simulink model "attempt_2_Full_Microthruster_Simulation"  (R2021b)
settings: Solver=ode45  StartTime=0.0  StopTime=simtime  RelTol=1e-16  AbsTol=1e-16
undefined symbols (not defined in the file): delta_t, dev_en, drag_unmodeled, dtype_g, euler_b_ECI0, euler_b_LVLH0, euler_LVLH_ECI0, g_bias, g_sath, g_satl, g_sen, g_sf_cc, geom, gr_eff_unmodeled, grav_grad_unmodeled, gyro_meas_frequ, J, JD_start, mag_field_unmodeled, mag_meas_frequ, mu, onboard_unmodeled, quat_b_ECI0, quat_b_LVLH0, quat_LVLH_ECI0, r, sigma_g, sigma_m, sigma_q, sigma_s, srp_unmodeled, sun_meas_frequ, theor_torque, ts, v, w_b_ECI0, wn, zn
libraries: aerolibnav x5, sharedTrackingLibrary x2
(part 2 of 2)

== matlab function attempt_2_Full_Microthruster_Simulation/Mag Sensor Measurement Function/MATLAB Function ==
  data: xk input; yy output; start_time input; sim_time input; sigma_m input; sigma_q input; posState input
function yy = h(xk,start_time,sim_time,sigma_m,sigma_q,posState)

yy = zeros([3 1]);
% Start time is initial juliandate
% Sim time is current sim time in seconds

JD_new = start_time + sim_time/3600/24; % add sim time in days to start time
t1 = datetime(JD_new,'ConvertFrom','juliandate');

q = xk(4:7);
eps = q(1:3);
eta = q(4);
r_ECI = posState(1:3);
[y, m, d] = ymd(t1);
[h, mm, s] = hms(t1);
utc_t1 = [y m d h mm s];
coder.extrinsic('eci2lla');
coder.extrinsic('igrfmagm');
coder.extrinsic('ned2ecefv');
coder.extrinsic('dcmeci2ecef');
coder.extrinsic('randn');
coder.extrinsic('decyear');

coder.extrinsic('Functions.Yb_func')
lla = eci2lla((r_ECI.*1e3)',utc_t1);
del = lla(1); % latitude
lambda = lla(2); % longitude
alt_g = lla(3);

% t = sim_time;
% % Set constants
% Re = 6378e3;                        % radius of the earth in m
% w_earth = 7.292e-5;                 % rad/s Earth rotation
% r_ECI_mag = norm(1e3.*r_ECI);       % magnitude of r ECI vector 
% m_b = [0;0;-0.5];                   % Residual magnetic dipole in body frame in A-m^2
% g1 = -29404.8*10^-9;                      % IGRF coeff constants
% g11 = -1450.9*10^-9;
% h11 = 4652.5*10^-9;

% Set intial conditions
% t0 = 0;                             % initial time

% Calculate B in BODY FRAME
% del = asin(r_ECI(3)/r_ECI_mag);     % geocentric latitude
% theta = pi/2 - del;                 % s/c geocentric co-latitude
% alpha = atan2((r_ECI(2)/sqrt(r_ECI(1)^2+r_ECI(2)^2)),... % s/c right ascension
%               (r_ECI(1)/sqrt(r_ECI(1)^2+r_ECI(2)^2))); 
% alpha_G = w_earth*(t-t0);           % right ascension of Greenwich meridian
% lambda = alpha - alpha_G;           % s/c geocentric longitude 
% C_ECI_s = Functions.Cz(-alpha)*Functions.Cy(del-pi/2);  % rotation matrix from spherical to ECI
% 
% mag_ECI = C_ECI_s*[2*(Re/r_ECI_mag)^3*(g1*cos(theta) + (g11*cos(lambda)+h11*sin(lambda))*sin(theta));
%          (Re/r_ECI_mag)^3*(g1*sin(theta) + (g11*cos(lambda)+h11*sin(lambda))*sin(theta));
%          (Re/r_ECI_mag)^3*(g11*sin(lambda) - h11*cos(lambda))]; % Earth magnetic field in spherical coordinates

igrf_m_NED = igrfmagm(alt_g,del,lambda,decyear(y,m,d))*1e-9;
igrf_m_ECEF = [0 0 0];
[igrf_m_ECEF(1),igrf_m_ECEF(2),igrf_m_ECEF(3)] = ned2ecefv(igrf_m_NED(1),igrf_m_NED(2),igrf_m_NED(3),del,lambda);

C_ECEF_ECI = dcmeci2ecef('IAU-2000/2006',utc_t1);
C_ECI_ECEF = C_ECEF_ECI';
mag_ECI = C_ECI_ECEF*igrf_m_ECEF';

% Calculate Y(a,q) for magnetometer and sun sensor


Y_b = Functions.Yb_func(q,mag_ECI);

v_k = zeros([3 1]); %#ok<*PREALL> simulink needs this to determine variable size
v_k = randn(3,1)*sigma_q;   
m_k = zeros([3 1]);
m_k = randn(3,1)*sigma_m;
% y = [zeros(3) Y_s]*xk + m_k + v_k; % measurement with measurement and process noise
% y = [zeros(3) Y_s]*xk + mk + v_k; % measurement with measurement and process noise
yy = [zeros(3) Y_b]*xk; % measurement with no noise

== matlab function attempt_2_Full_Microthruster_Simulation/Magnetometer ==
  data: xk input; JD_start input; yy output; sigma_m input; sigma_q input; sim_time input; posState input; yy_no_noise output
function [yy,yy_no_noise] = magVec(xk,JD_start,sigma_m,sigma_q,sim_time,posState)

yy = zeros([3 1]);
JD_new = JD_start + sim_time/3600/24; % add sim time in days to start time
t1 = datetime(JD_new,'ConvertFrom','juliandate');

q = xk(4:7);

r_ECI = posState(1:3);

[y, m, d] = ymd(t1);
[h, mm, s] = hms(t1);
utc_t1 = [y m d h mm s];

coder.extrinsic('eci2lla');
coder.extrinsic('igrfmagm');
coder.extrinsic('ned2ecefv');
coder.extrinsic('dcmeci2ecef');
coder.extrinsic('randn');
coder.extrinsic('decyear');
coder.extrinsic('Functions.Yb_func')
lla = eci2lla((r_ECI.*1e3)',utc_t1);
del = lla(1); % latitude
lambda = lla(2); % longitude
alt_g = lla(3);

% Set constants
% Re = 6378e3;                        % radius of the earth in m
% w_earth = 7.292e-5;                 % rad/s Earth rotation
% r_ECI_mag = norm(1e3.*r_ECI);       % magnitude of r ECI vector 
% m_b = [0;0;-0.5];                   % Residual magnetic dipole in body frame in A-m^2
% g1 = -29404.8*10^-9;                      % IGRF coeff constants
% g11 = -1450.9*10^-9;
% h11 = 4652.5*10^-9;

% Set intial conditions
% t0 = 0;                             % initial time

% Calculate B in BODY FRAME
% del = asin(r_ECI(3)/r_ECI_mag);     % geocentric latitude
% theta = pi/2 - del;                 % s/c geocentric co-latitude
% alpha = atan2((r_ECI(2)/sqrt(r_ECI(1)^2+r_ECI(2)^2)),... % s/c right ascension
%               (r_ECI(1)/sqrt(r_ECI(1)^2+r_ECI(2)^2))); 
% alpha_G = w_earth*(t-t0);           % right ascension of Greenwich meridian
% lambda = alpha - alpha_G;           % s/c geocentric longitude 
% C_ECI_s = Functions.Cz(-alpha)*Functions.Cy(del-pi/2);  % rotation matrix from spherical to ECI
% 
% mag_ECI = C_ECI_s*[2*(Re/r_ECI_mag)^3*(g1*cos(theta) + (g11*cos(lambda)+h11*sin(lambda))*sin(theta));
%          (Re/r_ECI_mag)^3*(g1*sin(theta) + (g11*cos(lambda)+h11*sin(lambda))*sin(theta));
%          (Re/r_ECI_mag)^3*(g11*sin(lambda) - h11*cos(lambda))]; % Earth magnetic field in spherical coordinates

igrf_m_NED = igrfmagm(alt_g,del,lambda,decyear(y,m,d))*1e-9;
igrf_m_ECEF = [0 0 0];
[igrf_m_ECEF(1),igrf_m_ECEF(2),igrf_m_ECEF(3)] = ned2ecefv(igrf_m_NED(1),igrf_m_NED(2),igrf_m_NED(3),del,lambda);

C_ECEF_ECI = dcmeci2ecef('IAU-2000/2006',utc_t1);
C_ECI_ECEF = C_ECEF_ECI';
mag_ECI = [0;0;0];
mag_ECI = C_ECI_ECEF*igrf_m_ECEF';

% Calculate Y(a,q) for magnetometer and sun sensor
Y_b = zeros([3 4]);
Y_b = Functions.Yb_func(q,mag_ECI);
% Y_b = [eta*eye(3)-vec2cross(eps) -eps]*[Functions.vec2cross(mag_ECI) mag_ECI;
%                                                       -mag_ECI'                    0];
% Y_s = [eta*eye(3)-Functions.vec2cross(eps) -eps]*[Functions.vec2cross(sun_ECI) sun_ECI;
%                                                       -sun_ECI'                    0];

v_k = zeros([3 1]); %#ok<*PREALL> simulink needs this to determine variable size
v_k = randn(3,1)*sigma_q;   
m_k = zeros([3 1]);
m_k = [randn(3,1)*sigma_m];
yy_no_noise = [zeros(3) Y_b]*xk;
yy = yy_no_noise + m_k; % measurement with measurement and process noise
% y = [zeros(3) Y_s]*xk; % measurement with no noise

== matlab function attempt_2_Full_Microthruster_Simulation/State Transition Function/Perturbation Model 2/B Field/MATLAB Function ==
  data: state_rb input; Tmb output; attState input; t input
function Tmb = fcn(state_rb,attState,t)

%%% MAGNETIC FIELD %%%%%
r_ECI = state_rb(1:3)';
      
q = attState(4:end); % extract quaternion from attitude state
C_b_ECI = Functions.quat2rot(q); % get ECI to BODY rotation matrix % turn r_ECI into a column vector

% Set constants
Re = 6378e3;                        % radius of the earth in m
w_earth = 7.292e-5;                 % rad/s Earth rotation
r_ECI_mag = norm(1e3.*r_ECI);       % magnitude of r ECI vector 
m_b = [0;0;-0.5];                   % Residual magnetic dipole in body frame in A-m^2
g1 = -29404.8*10^-9;                      % IGRF coeff constants
g11 = -1450.9*10^-9;
h11 = 4652.5*10^-9;

% Set intial conditions
t0 = 0;                             % initial time

% Calculate B in BODY FRAME
del = asin(r_ECI(3)/r_ECI_mag);     % geocentric latitude
theta = pi/2 - del;                 % s/c geocentric co-latitude
alpha = atan2((r_ECI(2)/sqrt(r_ECI(1)^2+r_ECI(2)^2)),... % s/c right ascension
              (r_ECI(1)/sqrt(r_ECI(1)^2+r_ECI(2)^2))); 
alpha_G = w_earth*(t-t0);           % right ascension of Greenwich meridian
lambda = alpha - alpha_G;           % s/c geocentric longitude 
C_ECI_s = Functions.Cz(-alpha)*Functions.Cy(del-pi/2);  % rotation matrix from spherical to ECI

B_s = [2*(Re/r_ECI_mag)^3*(g1*cos(theta) + (g11*cos(lambda)+h11*sin(lambda))*sin(theta));
         (Re/r_ECI_mag)^3*(g1*sin(theta) + (g11*cos(lambda)+h11*sin(lambda))*sin(theta));
         (Re/r_ECI_mag)^3*(g11*sin(lambda) - h11*cos(lambda))]; % Earth magnetic field in spherical coordinates

B_b = C_b_ECI*C_ECI_s*B_s;          % Earth magnetic field in BODY frame
Tmb = [0;0;0];
Tmb = cross(m_b,B_b);               % magnetic field torque

== matlab function attempt_2_Full_Microthruster_Simulation/State Transition Function/Perturbation Model 2/Drag/MATLAB Function ==
  data: state input; Td output; attState input; geom input
function Td = fcn(state,attState,geom)

% Extract s/c geometry parameters
x = geom(1); % x-axis
y = geom(3); % y-axis
z = geom(2); % z-axis

v_ECI = state(4:6);
   
q = attState(4:end); % extract quaternion from attitude state
C_b_ECI = Functions.quat2rot(q);                 % get ECI to BODY rotation matrix 

%%%%%% ATMO DRAG %%%%%%%
v_b = 1000.*(C_b_ECI*v_ECI);    % velocity vector in BODY frame
v_mag = norm(v_b);      % velocity vector magnitude BODY frame
v_dir = v_b./v_mag;     % velocity unit vector BODY frame
Cd = 2.2;               % approximate coefficent of drag
rho = 1.49e-15;        % km/m^3 US std atmosphere


Ta = [0;0;0];                    % Initialzie atmo torque vector
Fd_coeff = -1/2*rho*v_mag^2*Cd;  % Calculate constant coeff for speed

% Instantiate CoP vectors
CoM_vec = [0;0;0]; % From mass_props inertia calculations; assume CoM is at center of body frame

%%%%%%%%%BUS COP VECTORS%%%%%%%%%%%%%%%%
BUS_neg_z = [0;0;-z/2];
CP_BUS_neg_z = CoM_vec - BUS_neg_z;

BUS_pos_z = -BUS_neg_z;
CP_BUS_pos_z = CoM_vec - BUS_pos_z;

BUS_neg_y = [0;-y/2;0];
CP_BUS_neg_y = CoM_vec - BUS_neg_y;

BUS_pos_y = -BUS_neg_y;
CP_BUS_pos_y = CoM_vec - BUS_pos_y;

BUS_neg_x = [-x/2;0;0];
CP_BUS_neg_x = CoM_vec - BUS_neg_x;

BUS_pos_x = -BUS_neg_x;
CP_BUS_pos_x = CoM_vec - BUS_pos_x;

% Find area of each exposed surface
A_SP_y_side = x*z;
A_SP_x_side = y*z;
A_SP_z_side = x*y;

% Create normal directional vectors
x_dir = [1;0;0];
y_dir = [0;1;0];
z_dir = [0;0;1];
dir_vector = {x_dir,-x_dir,y_dir,-y_dir,z_dir,-z_dir};

% Create arrays of areas and CoM-->CoP vectors for each surface for each
% normal direction (x, -x, y, -y, z, -z)
pos_x_COP_vectors = [CP_BUS_pos_x];
pos_x_areas       = [A_SP_x_side];

neg_x_areas        = pos_x_areas;
neg_x_COP_vectors = [CP_BUS_neg_x];

pos_y_COP_vectors = [CP_BUS_pos_y];
pos_y_areas        = [A_SP_y_side];

neg_y_areas        = pos_y_areas;
neg_y_COP_vectors = [CP_BUS_neg_y];

neg_z_areas        = [A_SP_z_side];
neg_z_COP_vectors = [CP_BUS_neg_z];

pos_z_areas        = [A_SP_z_side];
pos_z_COP_vectors = [CP_BUS_pos_z];

% Combine cell arrays of area and their corresponding vectors into parent
% cell arrays
CoP_vectors = {pos_x_COP_vectors,neg_x_COP_vectors,...
               pos_y_COP_vectors,neg_y_COP_vectors,...
               pos_z_COP_vectors,neg_z_COP_vectors};
areas = {pos_x_areas,neg_x_areas,pos_y_areas,neg_y_areas,pos_z_areas,neg_z_areas};

for i = 1:length(dir_vector)
    dire = dir_vector{i};
    if dot(dire,v_dir) >= 0
        curr_area = areas{i};
        curr_CoP_vec = CoP_vectors{i};
        for ii = 1:length(curr_area)
            Fd = dot(dire,v_dir)*Fd_coeff*curr_area(ii).*v_dir;
            Ta = Ta + cross(curr_CoP_vec(:,ii),Fd);
        end
    end
end

Td= Ta;

== matlab function attempt_2_Full_Microthruster_Simulation/State Transition Function/Perturbation Model 2/Gravity Gradient/MATLAB Function ==
  data: J input; Tgg output; state_rb input; attState input
function Tgg = fcn(J,state_rb,attState)

q = attState(4:end); % extract quaternion from attitude state

r_ECI = state_rb(1:3)*1000;
mu = 398600*1000^3;
   
C_b_ECI = Functions.quat2rot(q); % get ECI to BODY rotation matrix % turn r_ECI into a column vector
r_b = C_b_ECI*r_ECI;                        % Get r in terms of BODY frame
r_mag = norm(r_b);                          % Get magnitude of r in BODY frame
Tgg = (3*mu/r_mag^5)*Functions.vec2cross(r_b)*J*r_b; % Gravity gradient calculation

== matlab function attempt_2_Full_Microthruster_Simulation/State Transition Function/Perturbation Model 2/SRP/MATLAB Function ==
  data: attState input; Tsrp output; geom input
function Tsrp = fcn(attState,geom)


% Extract s/c geometry parameters
x = geom(1); % x-axis
y = geom(3); % y-axis
z = geom(2); % z-axis


q = attState(4:end); % extract quaternion from attitude state
C_b_ECI = Functions.quat2rot(q);                 % get ECI to BODY rotation matrix 
s_dir = C_b_ECI*[-1;0;0];     % solar radiation pressure unit vector BODY frame

%%%%%% ATMO DRAG %%%%%%%

% Instantiate CoP vectors
CoM_vec = [0;0;0]; % From mass_props inertia calculations; assume CoM is at center of body frame

%%%%%%%%%BUS COP VECTORS%%%%%%%%%%%%%%%%
BUS_neg_z = [0;0;-z/2];
CP_BUS_neg_z = CoM_vec - BUS_neg_z;

BUS_pos_z = -BUS_neg_z;
CP_BUS_pos_z = CoM_vec - BUS_pos_z;

BUS_neg_y = [0;-y/2;0];
CP_BUS_neg_y = CoM_vec - BUS_neg_y;

BUS_pos_y = -BUS_neg_y;
CP_BUS_pos_y = CoM_vec - BUS_pos_y;

BUS_neg_x = [-x/2;0;0];
CP_BUS_neg_x = CoM_vec - BUS_neg_x;

BUS_pos_x = -BUS_neg_x;
CP_BUS_pos_x = CoM_vec - BUS_pos_x;

% Find area of each exposed surface
A_SP_y_side = x*z;
A_SP_x_side = y*z;
A_SP_z_side = x*y;

% Create normal directional vectors
x_dir = [1;0;0];
y_dir = [0;1;0];
z_dir = [0;0;1];
dir_vector = {x_dir,-x_dir,y_dir,-y_dir,z_dir,-z_dir};

% Create arrays of areas and CoM-->CoP vectors for each surface for each
% normal direction (x, -x, y, -y, z, -z)
pos_x_COP_vectors = [CP_BUS_pos_x];
pos_x_areas       = [A_SP_x_side];

neg_x_areas        = pos_x_areas;
neg_x_COP_vectors = [CP_BUS_neg_x];

pos_y_COP_vectors = [CP_BUS_pos_y];
pos_y_areas        = [A_SP_y_side];

neg_y_areas        = pos_y_areas;
neg_y_COP_vectors = [CP_BUS_neg_y];

neg_z_areas        = [A_SP_z_side];
neg_z_COP_vectors = [CP_BUS_neg_z];

pos_z_areas        = [A_SP_z_side];
pos_z_COP_vectors = [CP_BUS_pos_z];

% Combine cell arrays of area and their corresponding vectors into parent
% cell arrays
CoP_vectors = {pos_x_COP_vectors,neg_x_COP_vectors,...
               pos_y_COP_vectors,neg_y_COP_vectors,...
               pos_z_COP_vectors,neg_z_COP_vectors};
areas = {pos_x_areas,neg_x_areas,pos_y_areas,neg_y_areas,pos_z_areas,neg_z_areas};

p_s = 4.5e-06; % solar const N/m^2
Tsrp = [0;0;0];                    % Initialzie atmo torque vector
for i = 1:length(dir_vector)
    dire = dir_vector{i};
    if dot(dire,s_dir) > 0
        curr_area = areas{i};
        curr_CoP_vec = CoP_vectors{i};
        for ii = 1:length(curr_area)
            Fs = -dot(dire,s_dir)*p_s*curr_area(ii).*s_dir;
            Tsrp = Tsrp + cross(curr_CoP_vec(:,ii),Fs);
        end
    end
end

== matlab function attempt_2_Full_Microthruster_Simulation/State Transition Function/MATLAB Function ==
  data: x_k_1 input; x_k output; u_k_1 input; T_thrust input; T_other input; J input; Ts input
function x_k = f(x_k_1,u_k_1,T_thrust,T_other,J,Ts)
% State transition function; propogating state (angular velocity and
% quaternion column vector) to new state via regular dynamic equations
% u_k_1 is some "control" value; set to 0 here
omega_k_1 = x_k_1(1:3);
quat_k_1 = x_k_1(4:7);

% Get last step b_ECI rotation matrix
C_b_ECI = Functions.quat2rot(quat_k_1);

% Turn given thrust vector from body to ECI
T_thrust = C_b_ECI'*T_thrust; % transpose b_ECI to get body->ECI rot matrix

T = T_thrust + T_other; % sum considered control/perturbation torques with applied thrust

eps = quat_k_1(1:3);
eta = quat_k_1(4);

x_k = x_k_1 + Ts*[J\(T-Functions.vec2cross(omega_k_1)*J*omega_k_1 + u_k_1);
                 0.5*(eta*eye(3)+Functions.vec2cross(eps))*omega_k_1;
                -0.5*eps'*omega_k_1];

== matlab function attempt_2_Full_Microthruster_Simulation/Mag Sensor Measurement Function1/MATLAB Function ==
  data: xk input; JD_start input; yy output; sim_time input; sigma_m input; sigma_q input; posState input
function yy = h(xk,JD_start,sim_time,sigma_m,sigma_q,posState)

% Start time is initial juliandate
% Sim time is current sim time in seconds

yy = zeros([3 1]);
JD_new = JD_start + sim_time/3600/24; % add sim time in days to start time
t1 = datetime(JD_new,'ConvertFrom','juliandate');

q = xk(4:7);
eps = q(1:3);
eta = q(4);
r_ECI = posState(1:3);
[y, m, d] = ymd(t1);
[h, mm, s] = hms(t1);
utc_t1 = [y m d h mm s];
coder.extrinsic('eci2lla');
coder.extrinsic('igrfmagm');
coder.extrinsic('ned2ecefv');
coder.extrinsic('dcmeci2ecef');
coder.extrinsic('randn');
coder.extrinsic('decyear');

coder.extrinsic('Functions.Yb_func')
lla = eci2lla((r_ECI.*1e3)',utc_t1);
del = lla(1); % latitude
lambda = lla(2); % longitude
alt_g = lla(3);

% t = sim_time;
% % Set constants
% Re = 6378e3;                        % radius of the earth in m
% w_earth = 7.292e-5;                 % rad/s Earth rotation
% r_ECI_mag = norm(1e3.*r_ECI);       % magnitude of r ECI vector 
% m_b = [0;0;-0.5];                   % Residual magnetic dipole in body frame in A-m^2
% g1 = -29404.8*10^-9;                      % IGRF coeff constants
% g11 = -1450.9*10^-9;
% h11 = 4652.5*10^-9;

% Set intial conditions
% t0 = 0;                             % initial time

% Calculate B in BODY FRAME
% del = asin(r_ECI(3)/r_ECI_mag);     % geocentric latitude
% theta = pi/2 - del;                 % s/c geocentric co-latitude
% alpha = atan2((r_ECI(2)/sqrt(r_ECI(1)^2+r_ECI(2)^2)),... % s/c right ascension
%               (r_ECI(1)/sqrt(r_ECI(1)^2+r_ECI(2)^2))); 
% alpha_G = w_earth*(t-t0);           % right ascension of Greenwich meridian
% lambda = alpha - alpha_G;           % s/c geocentric longitude 
% C_ECI_s = Functions.Cz(-alpha)*Functions.Cy(del-pi/2);  % rotation matrix from spherical to ECI
% 
% mag_ECI = C_ECI_s*[2*(Re/r_ECI_mag)^3*(g1*cos(theta) + (g11*cos(lambda)+h11*sin(lambda))*sin(theta));
%          (Re/r_ECI_mag)^3*(g1*sin(theta) + (g11*cos(lambda)+h11*sin(lambda))*sin(theta));
%          (Re/r_ECI_mag)^3*(g11*sin(lambda) - h11*cos(lambda))]; % Earth magnetic field in spherical coordinates

igrf_m_NED = igrfmagm(alt_g,del,lambda,decyear(y,m,d))*1e-9;
igrf_m_ECEF = [0 0 0];
[igrf_m_ECEF(1),igrf_m_ECEF(2),igrf_m_ECEF(3)] = ned2ecefv(igrf_m_NED(1),igrf_m_NED(2),igrf_m_NED(3),del,lambda);

C_ECEF_ECI = dcmeci2ecef('IAU-2000/2006',utc_t1);
C_ECI_ECEF = C_ECEF_ECI';
mag_ECI = C_ECI_ECEF*igrf_m_ECEF';

% Calculate Y(a,q) for magnetometer and sun sensor

Y_b = Functions.Yb_func(q,mag_ECI);

v_k = zeros([3 1]); %#ok<*PREALL> simulink needs this to determine variable size
v_k = randn(3,1)*sigma_q;   
m_k = zeros([3 1]);
m_k = randn(3,1)*sigma_m;
% y = [zeros(3) Y_s]*xk + m_k + v_k; % measurement with measurement and process noise
% y = [zeros(3) Y_s]*xk + mk + v_k; % measurement with measurement and process noise
yy = [zeros(3) Y_b]*xk; % measurement with no noise

== matlab function attempt_2_Full_Microthruster_Simulation/State Transition Function1/MATLAB Function ==
  data: x_k_1 input; x_k output; u_k_1 input; T_thrust input; T_other input; J input; Ts input
function x_k = f(x_k_1,u_k_1,T_thrust,T_other,J,Ts)
% State transition function; propogating state (angular velocity and
% quaternion column vector) to new state via regular dynamic equations
% u_k_1 is some "control" value; set to 0 here
omega_k_1 = x_k_1(1:3);
quat_k_1 = x_k_1(4:7);

% Get last step b_ECI rotation matrix
C_b_ECI = Functions.quat2rot(quat_k_1);

% Turn given thrust vector from body to ECI
T_thrust = C_b_ECI'*T_thrust; % transpose b_ECI to get body->ECI rot matrix

T = T_thrust + T_other; % sum considered control/perturbation torques with applied thrust

eps = quat_k_1(1:3);
eta = quat_k_1(4);

x_k = x_k_1 + Ts*[J\(T-Functions.vec2cross(omega_k_1)*J*omega_k_1 + u_k_1);
                 0.5*(eta*eye(3)+Functions.vec2cross(eps))*omega_k_1;
                -0.5*eps'*omega_k_1];

== matlab function attempt_2_Full_Microthruster_Simulation/State Transition Function1/Perturbation Model 2/B Field/MATLAB Function ==
  data: state_rb input; Tmb output; attState input; t input
function Tmb = fcn(state_rb,attState,t)

%%% MAGNETIC FIELD %%%%%
r_ECI = state_rb(1:3)';
      
q = attState(4:end); % extract quaternion from attitude state
C_b_ECI = Functions.quat2rot(q); % get ECI to BODY rotation matrix % turn r_ECI into a column vector

% Set constants
Re = 6378e3;                        % radius of the earth in m
w_earth = 7.292e-5;                 % rad/s Earth rotation
r_ECI_mag = norm(1e3.*r_ECI);       % magnitude of r ECI vector 
m_b = [0;0;-0.5];                   % Residual magnetic dipole in body frame in A-m^2
g1 = -29404.8*10^-9;                      % IGRF coeff constants
g11 = -1450.9*10^-9;
h11 = 4652.5*10^-9;

% Set intial conditions
t0 = 0;                             % initial time

% Calculate B in BODY FRAME
del = asin(r_ECI(3)/r_ECI_mag);     % geocentric latitude
theta = pi/2 - del;                 % s/c geocentric co-latitude
alpha = atan2((r_ECI(2)/sqrt(r_ECI(1)^2+r_ECI(2)^2)),... % s/c right ascension
              (r_ECI(1)/sqrt(r_ECI(1)^2+r_ECI(2)^2))); 
alpha_G = w_earth*(t-t0);           % right ascension of Greenwich meridian
lambda = alpha - alpha_G;           % s/c geocentric longitude 
C_ECI_s = Functions.Cz(-alpha)*Functions.Cy(del-pi/2);  % rotation matrix from spherical to ECI

B_s = [2*(Re/r_ECI_mag)^3*(g1*cos(theta) + (g11*cos(lambda)+h11*sin(lambda))*sin(theta));
         (Re/r_ECI_mag)^3*(g1*sin(theta) + (g11*cos(lambda)+h11*sin(lambda))*sin(theta));
         (Re/r_ECI_mag)^3*(g11*sin(lambda) - h11*cos(lambda))]; % Earth magnetic field in spherical coordinates

B_b = C_b_ECI*C_ECI_s*B_s;          % Earth magnetic field in BODY frame
Tmb = [0;0;0];
Tmb = cross(m_b,B_b);               % magnetic field torque

== matlab function attempt_2_Full_Microthruster_Simulation/State Transition Function1/Perturbation Model 2/Drag/MATLAB Function ==
  data: state input; Td output; attState input; geom input
function Td = fcn(state,attState,geom)

% Extract s/c geometry parameters
x = geom(1); % x-axis
y = geom(3); % y-axis
z = geom(2); % z-axis

v_ECI = state(4:6);
   
q = attState(4:end); % extract quaternion from attitude state
C_b_ECI = Functions.quat2rot(q);                 % get ECI to BODY rotation matrix 

%%%%%% ATMO DRAG %%%%%%%
v_b = 1000.*(C_b_ECI*v_ECI);    % velocity vector in BODY frame
v_mag = norm(v_b);      % velocity vector magnitude BODY frame
v_dir = v_b./v_mag;     % velocity unit vector BODY frame
Cd = 2.2;               % approximate coefficent of drag
rho = 1.49e-15;        % km/m^3 US std atmosphere


Ta = [0;0;0];                    % Initialzie atmo torque vector
Fd_coeff = -1/2*rho*v_mag^2*Cd;  % Calculate constant coeff for speed

% Instantiate CoP vectors
CoM_vec = [0;0;0]; % From mass_props inertia calculations; assume CoM is at center of body frame

%%%%%%%%%BUS COP VECTORS%%%%%%%%%%%%%%%%
BUS_neg_z = [0;0;-z/2];
CP_BUS_neg_z = CoM_vec - BUS_neg_z;

BUS_pos_z = -BUS_neg_z;
CP_BUS_pos_z = CoM_vec - BUS_pos_z;

BUS_neg_y = [0;-y/2;0];
CP_BUS_neg_y = CoM_vec - BUS_neg_y;

BUS_pos_y = -BUS_neg_y;
CP_BUS_pos_y = CoM_vec - BUS_pos_y;

BUS_neg_x = [-x/2;0;0];
CP_BUS_neg_x = CoM_vec - BUS_neg_x;

BUS_pos_x = -BUS_neg_x;
CP_BUS_pos_x = CoM_vec - BUS_pos_x;

% Find area of each exposed surface
A_SP_y_side = x*z;
A_SP_x_side = y*z;
A_SP_z_side = x*y;

% Create normal directional vectors
x_dir = [1;0;0];
y_dir = [0;1;0];
z_dir = [0;0;1];
dir_vector = {x_dir,-x_dir,y_dir,-y_dir,z_dir,-z_dir};

% Create arrays of areas and CoM-->CoP vectors for each surface for each
% normal direction (x, -x, y, -y, z, -z)
pos_x_COP_vectors = [CP_BUS_pos_x];
pos_x_areas       = [A_SP_x_side];

neg_x_areas        = pos_x_areas;
neg_x_COP_vectors = [CP_BUS_neg_x];

pos_y_COP_vectors = [CP_BUS_pos_y];
pos_y_areas        = [A_SP_y_side];

neg_y_areas        = pos_y_areas;
neg_y_COP_vectors = [CP_BUS_neg_y];

neg_z_areas        = [A_SP_z_side];
neg_z_COP_vectors = [CP_BUS_neg_z];

pos_z_areas        = [A_SP_z_side];
pos_z_COP_vectors = [CP_BUS_pos_z];

% Combine cell arrays of area and their corresponding vectors into parent
% cell arrays
CoP_vectors = {pos_x_COP_vectors,neg_x_COP_vectors,...
               pos_y_COP_vectors,neg_y_COP_vectors,...
               pos_z_COP_vectors,neg_z_COP_vectors};
areas = {pos_x_areas,neg_x_areas,pos_y_areas,neg_y_areas,pos_z_areas,neg_z_areas};

for i = 1:length(dir_vector)
    dire = dir_vector{i};
    if dot(dire,v_dir) >= 0
        curr_area = areas{i};
        curr_CoP_vec = CoP_vectors{i};
        for ii = 1:length(curr_area)
            Fd = dot(dire,v_dir)*Fd_coeff*curr_area(ii).*v_dir;
            Ta = Ta + cross(curr_CoP_vec(:,ii),Fd);
        end
    end
end

Td= Ta;

== matlab function attempt_2_Full_Microthruster_Simulation/Orbital Motion Propagator/MATLAB Function ==
  data: T input; Tt input; Tu input; I input; domega output; omega input; domega_thrust output
function [domega, domega_thrust] = DYNAMICS(T,Tt,Tu,I,omega)

Ttot = T+Tt+Tu;
domega = I\(Ttot-Functions.vec2cross(omega)*I*omega);

domega_thrust = I\(Tt-Functions.vec2cross(omega)*I*omega);
% domega = I\(T-cross(omega,I*omega));

end

== matlab function attempt_2_Full_Microthruster_Simulation/Perturbation Model 2/B Field/MATLAB Function ==
  data: state_rb input; Tmb output; attState input; t input
function Tmb = fcn(state_rb,attState,t)

%%% MAGNETIC FIELD %%%%%
r_ECI = state_rb(1:3)';
      
q = attState(4:end); % extract quaternion from attitude state
C_b_ECI = Functions.quat2rot(q); % get ECI to BODY rotation matrix % turn r_ECI into a column vector

% Set constants
Re = 6378e3;                        % radius of the earth in m
w_earth = 7.292e-5;                 % rad/s Earth rotation
r_ECI_mag = norm(1e3.*r_ECI);       % magnitude of r ECI vector 
m_b = [0;0;-0.5];                   % Residual magnetic dipole in body frame in A-m^2
g1 = -29404.8*10^-9;                      % IGRF coeff constants
g11 = -1450.9*10^-9;
h11 = 4652.5*10^-9;

% Set intial conditions
t0 = 0;                             % initial time

% Calculate B in BODY FRAME
del = asin(r_ECI(3)/r_ECI_mag);     % geocentric latitude
theta = pi/2 - del;                 % s/c geocentric co-latitude
alpha = atan2((r_ECI(2)/sqrt(r_ECI(1)^2+r_ECI(2)^2)),... % s/c right ascension
              (r_ECI(1)/sqrt(r_ECI(1)^2+r_ECI(2)^2))); 
alpha_G = w_earth*(t-t0);           % right ascension of Greenwich meridian
lambda = alpha - alpha_G;           % s/c geocentric longitude 
C_ECI_s = Functions.Cz(-alpha)*Functions.Cy(del-pi/2);  % rotation matrix from spherical to ECI

B_s = [2*(Re/r_ECI_mag)^3*(g1*cos(theta) + (g11*cos(lambda)+h11*sin(lambda))*sin(theta));
         (Re/r_ECI_mag)^3*(g1*sin(theta) + (g11*cos(lambda)+h11*sin(lambda))*sin(theta));
         (Re/r_ECI_mag)^3*(g11*sin(lambda) - h11*cos(lambda))]; % Earth magnetic field in spherical coordinates

B_b = C_b_ECI*C_ECI_s*B_s;          % Earth magnetic field in BODY frame
Tmb = [0;0;0];
Tmb = cross(m_b,B_b);               % magnetic field torque

== matlab function attempt_2_Full_Microthruster_Simulation/Perturbation Model 2/Drag/MATLAB Function ==
  data: state input; Td output; attState input; geom input
function Td = fcn(state,attState,geom)

% Extract s/c geometry parameters
x = geom(1); % x-axis
y = geom(3); % y-axis
z = geom(2); % z-axis

v_ECI = state(4:6);
   
q = attState(4:end); % extract quaternion from attitude state
C_b_ECI = Functions.quat2rot(q);                 % get ECI to BODY rotation matrix 

%%%%%% ATMO DRAG %%%%%%%
v_b = 1000.*(C_b_ECI*v_ECI);    % velocity vector in BODY frame
v_mag = norm(v_b);      % velocity vector magnitude BODY frame
v_dir = v_b./v_mag;     % velocity unit vector BODY frame
Cd = 2.2;               % approximate coefficent of drag
rho = 1.49e-15;        % km/m^3 US std atmosphere


Ta = [0;0;0];                    % Initialzie atmo torque vector
Fd_coeff = -1/2*rho*v_mag^2*Cd;  % Calculate constant coeff for speed

% Instantiate CoP vectors
CoM_vec = [0;0;0]; % From mass_props inertia calculations; assume CoM is at center of body frame

%%%%%%%%%BUS COP VECTORS%%%%%%%%%%%%%%%%
BUS_neg_z = [0;0;-z/2];
CP_BUS_neg_z = CoM_vec - BUS_neg_z;

BUS_pos_z = -BUS_neg_z;
CP_BUS_pos_z = CoM_vec - BUS_pos_z;

BUS_neg_y = [0;-y/2;0];
CP_BUS_neg_y = CoM_vec - BUS_neg_y;

BUS_pos_y = -BUS_neg_y;
CP_BUS_pos_y = CoM_vec - BUS_pos_y;

BUS_neg_x = [-x/2;0;0];
CP_BUS_neg_x = CoM_vec - BUS_neg_x;

BUS_pos_x = -BUS_neg_x;
CP_BUS_pos_x = CoM_vec - BUS_pos_x;

% Find area of each exposed surface
A_SP_y_side = x*z;
A_SP_x_side = y*z;
A_SP_z_side = x*y;

% Create normal directional vectors
x_dir = [1;0;0];
y_dir = [0;1;0];
z_dir = [0;0;1];
dir_vector = {x_dir,-x_dir,y_dir,-y_dir,z_dir,-z_dir};

% Create arrays of areas and CoM-->CoP vectors for each surface for each
% normal direction (x, -x, y, -y, z, -z)
pos_x_COP_vectors = [CP_BUS_pos_x];
pos_x_areas       = [A_SP_x_side];

neg_x_areas        = pos_x_areas;
neg_x_COP_vectors = [CP_BUS_neg_x];

pos_y_COP_vectors = [CP_BUS_pos_y];
pos_y_areas        = [A_SP_y_side];

neg_y_areas        = pos_y_areas;
neg_y_COP_vectors = [CP_BUS_neg_y];

neg_z_areas        = [A_SP_z_side];
neg_z_COP_vectors = [CP_BUS_neg_z];

pos_z_areas        = [A_SP_z_side];
pos_z_COP_vectors = [CP_BUS_pos_z];

% Combine cell arrays of area and their corresponding vectors into parent
% cell arrays
CoP_vectors = {pos_x_COP_vectors,neg_x_COP_vectors,...
               pos_y_COP_vectors,neg_y_COP_vectors,...
               pos_z_COP_vectors,neg_z_COP_vectors};
areas = {pos_x_areas,neg_x_areas,pos_y_areas,neg_y_areas,pos_z_areas,neg_z_areas};

for i = 1:length(dir_vector)
    dire = dir_vector{i};
    if dot(dire,v_dir) >= 0
        curr_area = areas{i};
        curr_CoP_vec = CoP_vectors{i};
        for ii = 1:length(curr_area)
            Fd = dot(dire,v_dir)*Fd_coeff*curr_area(ii).*v_dir;
            Ta = Ta + cross(curr_CoP_vec(:,ii),Fd);
        end
    end
end

Td= Ta;

== matlab function attempt_2_Full_Microthruster_Simulation/Perturbation Model 2/Gravity Gradient/MATLAB Function ==
  data: J input; Tgg output; state_rb input; attState input
function Tgg = fcn(J,state_rb,attState)

q = attState(4:end); % extract quaternion from attitude state

r_ECI = state_rb(1:3)*1000;
mu = 398600*1000^3;
   
C_b_ECI = Functions.quat2rot(q); % get ECI to BODY rotation matrix % turn r_ECI into a column vector
r_b = C_b_ECI*r_ECI;                        % Get r in terms of BODY frame
r_mag = norm(r_b);                          % Get magnitude of r in BODY frame
Tgg = (3*mu/r_mag^5)*Functions.vec2cross(r_b)*J*r_b; % Gravity gradient calculation

== matlab function attempt_2_Full_Microthruster_Simulation/Perturbation Model 2/SRP/MATLAB Function ==
  data: attState input; Tsrp output; geom input
function Tsrp = fcn(attState,geom)


% Extract s/c geometry parameters
x = geom(1); % x-axis
y = geom(3); % y-axis
z = geom(2); % z-axis


q = attState(4:end); % extract quaternion from attitude state
C_b_ECI = Functions.quat2rot(q);                 % get ECI to BODY rotation matrix 
s_dir = C_b_ECI*[-1;0;0];     % solar radiation pressure unit vector BODY frame

%%%%%% ATMO DRAG %%%%%%%

% Instantiate CoP vectors
CoM_vec = [0;0;0]; % From mass_props inertia calculations; assume CoM is at center of body frame

%%%%%%%%%BUS COP VECTORS%%%%%%%%%%%%%%%%
BUS_neg_z = [0;0;-z/2];
CP_BUS_neg_z = CoM_vec - BUS_neg_z;

BUS_pos_z = -BUS_neg_z;
CP_BUS_pos_z = CoM_vec - BUS_pos_z;

BUS_neg_y = [0;-y/2;0];
CP_BUS_neg_y = CoM_vec - BUS_neg_y;

BUS_pos_y = -BUS_neg_y;
CP_BUS_pos_y = CoM_vec - BUS_pos_y;

BUS_neg_x = [-x/2;0;0];
CP_BUS_neg_x = CoM_vec - BUS_neg_x;

BUS_pos_x = -BUS_neg_x;
CP_BUS_pos_x = CoM_vec - BUS_pos_x;

% Find area of each exposed surface
A_SP_y_side = x*z;
A_SP_x_side = y*z;
A_SP_z_side = x*y;

% Create normal directional vectors
x_dir = [1;0;0];
y_dir = [0;1;0];
z_dir = [0;0;1];
dir_vector = {x_dir,-x_dir,y_dir,-y_dir,z_dir,-z_dir};

% Create arrays of areas and CoM-->CoP vectors for each surface for each
% normal direction (x, -x, y, -y, z, -z)
pos_x_COP_vectors = [CP_BUS_pos_x];
pos_x_areas       = [A_SP_x_side];

neg_x_areas        = pos_x_areas;
neg_x_COP_vectors = [CP_BUS_neg_x];

pos_y_COP_vectors = [CP_BUS_pos_y];
pos_y_areas        = [A_SP_y_side];

neg_y_areas        = pos_y_areas;
neg_y_COP_vectors = [CP_BUS_neg_y];

neg_z_areas        = [A_SP_z_side];
neg_z_COP_vectors = [CP_BUS_neg_z];

pos_z_areas        = [A_SP_z_side];
pos_z_COP_vectors = [CP_BUS_pos_z];

% Combine cell arrays of area and their corresponding vectors into parent
% cell arrays
CoP_vectors = {pos_x_COP_vectors,neg_x_COP_vectors,...
               pos_y_COP_vectors,neg_y_COP_vectors,...
               pos_z_COP_vectors,neg_z_COP_vectors};
areas = {pos_x_areas,neg_x_areas,pos_y_areas,neg_y_areas,pos_z_areas,neg_z_areas};

p_s = 4.5e-06; % solar const N/m^2
Tsrp = [0;0;0];                    % Initialzie atmo torque vector
for i = 1:length(dir_vector)
    dire = dir_vector{i};
    if dot(dire,s_dir) > 0
        curr_area = areas{i};
        curr_CoP_vec = CoP_vectors{i};
        for ii = 1:length(curr_area)
            Fs = -dot(dire,s_dir)*p_s*curr_area(ii).*s_dir;
            Tsrp = Tsrp + cross(curr_CoP_vec(:,ii),Fs);
        end
    end
end

== matlab function attempt_2_Full_Microthruster_Simulation/State Transition Function1/Perturbation Model 2/Gravity Gradient/MATLAB Function ==
  data: J input; Tgg output; state_rb input; attState input
function Tgg = fcn(J,state_rb,attState)

q = attState(4:end); % extract quaternion from attitude state

r_ECI = state_rb(1:3)*1000;
mu = 398600*1000^3;
   
C_b_ECI = Functions.quat2rot(q); % get ECI to BODY rotation matrix % turn r_ECI into a column vector
r_b = C_b_ECI*r_ECI;                        % Get r in terms of BODY frame
r_mag = norm(r_b);                          % Get magnitude of r in BODY frame
Tgg = (3*mu/r_mag^5)*Functions.vec2cross(r_b)*J*r_b; % Gravity gradient calculation

== matlab function attempt_2_Full_Microthruster_Simulation/State Transition Function1/Perturbation Model 2/SRP/MATLAB Function ==
  data: attState input; Tsrp output; geom input
function Tsrp = fcn(attState,geom)


% Extract s/c geometry parameters
x = geom(1); % x-axis
y = geom(3); % y-axis
z = geom(2); % z-axis


q = attState(4:end); % extract quaternion from attitude state
C_b_ECI = Functions.quat2rot(q);                 % get ECI to BODY rotation matrix 
s_dir = C_b_ECI*[-1;0;0];     % solar radiation pressure unit vector BODY frame

%%%%%% ATMO DRAG %%%%%%%

% Instantiate CoP vectors
CoM_vec = [0;0;0]; % From mass_props inertia calculations; assume CoM is at center of body frame

%%%%%%%%%BUS COP VECTORS%%%%%%%%%%%%%%%%
BUS_neg_z = [0;0;-z/2];
CP_BUS_neg_z = CoM_vec - BUS_neg_z;

BUS_pos_z = -BUS_neg_z;
CP_BUS_pos_z = CoM_vec - BUS_pos_z;

BUS_neg_y = [0;-y/2;0];
CP_BUS_neg_y = CoM_vec - BUS_neg_y;

BUS_pos_y = -BUS_neg_y;
CP_BUS_pos_y = CoM_vec - BUS_pos_y;

BUS_neg_x = [-x/2;0;0];
CP_BUS_neg_x = CoM_vec - BUS_neg_x;

BUS_pos_x = -BUS_neg_x;
CP_BUS_pos_x = CoM_vec - BUS_pos_x;

% Find area of each exposed surface
A_SP_y_side = x*z;
A_SP_x_side = y*z;
A_SP_z_side = x*y;

% Create normal directional vectors
x_dir = [1;0;0];
y_dir = [0;1;0];
z_dir = [0;0;1];
dir_vector = {x_dir,-x_dir,y_dir,-y_dir,z_dir,-z_dir};

% Create arrays of areas and CoM-->CoP vectors for each surface for each
% normal direction (x, -x, y, -y, z, -z)
pos_x_COP_vectors = [CP_BUS_pos_x];
pos_x_areas       = [A_SP_x_side];

neg_x_areas        = pos_x_areas;
neg_x_COP_vectors = [CP_BUS_neg_x];

pos_y_COP_vectors = [CP_BUS_pos_y];
pos_y_areas        = [A_SP_y_side];

neg_y_areas        = pos_y_areas;
neg_y_COP_vectors = [CP_BUS_neg_y];

neg_z_areas        = [A_SP_z_side];
neg_z_COP_vectors = [CP_BUS_neg_z];

pos_z_areas        = [A_SP_z_side];
pos_z_COP_vectors = [CP_BUS_pos_z];

% Combine cell arrays of area and their corresponding vectors into parent
% cell arrays
CoP_vectors = {pos_x_COP_vectors,neg_x_COP_vectors,...
               pos_y_COP_vectors,neg_y_COP_vectors,...
               pos_z_COP_vectors,neg_z_COP_vectors};
areas = {pos_x_areas,neg_x_areas,pos_y_areas,neg_y_areas,pos_z_areas,neg_z_areas};

p_s = 4.5e-06; % solar const N/m^2
Tsrp = [0;0;0];                    % Initialzie atmo torque vector
for i = 1:length(dir_vector)
    dire = dir_vector{i};
    if dot(dire,s_dir) > 0
        curr_area = areas{i};
        curr_CoP_vec = CoP_vectors{i};
        for ii = 1:length(curr_area)
            Fs = -dot(dire,s_dir)*p_s*curr_area(ii).*s_dir;
            Tsrp = Tsrp + cross(curr_CoP_vec(:,ii),Fs);
        end
    end
end

== matlab function attempt_2_Full_Microthruster_Simulation/Sun Sensor Measurement Function1/MATLAB Function ==
  data: xk input; y output; start_time input; sim_time input; sigma_s input; sigma_q input
function y = h(xk,start_time,sim_time,sigma_s,sigma_q)

% Start time is initial juliandate
% Sim time is current sim time in seconds

JD_new = start_time + sim_time/3600/24; % add sim time in days to start time

q = xk(4:7);
eps = q(1:3);
eta = q(4);

jul_cent = (JD_new-2451545)/36525; % julian centuries since 2000
lambda_S = wrapTo360(280.4606184 + 36000.77005361*jul_cent); % mean longitude of sun in deg
M_S = wrapTo360(357.5277233 + 35999.05034*jul_cent); % mean anomaly of sun in deg
lambda_e = wrapTo180(lambda_S + 1.914666471*sind(M_S) + 0.019994643*sind(2*M_S)); % ecliptic long of sun in deg

eps_sun = 23.439291-0.0130042*jul_cent;
sun_ECI = [cosd(lambda_e); cosd(eps_sun)*sind(lambda_e); sind(eps_sun)*sind(lambda_e)];

% Test for comparison
%sun_ECI = [1;0;0];
% Calculate Y(a,q) for magnetometer and sun sensor
% Y_b = [eta*eye(3)-Functions.vec2cross(eps) -eps]*[Functions.vec2cross(mag_ECI) mag_ECI;
%                                                       -mag_ECI'                    0];
Y_s = [eta*eye(3)-Functions.vec2cross(eps) -eps]*[Functions.vec2cross(sun_ECI) sun_ECI;
                                                      -sun_ECI'                    0];

coder.extrinsic('randn');
v_k = zeros([3 1]); %#ok<*PREALL> simulink needs this to determine variable size
v_k = randn(3,1)*sigma_q;   
m_k = zeros([3 1]);
m_k = randn(3,1)*sigma_s;
% y = [zeros(3) Y_s]*xk + m_k + v_k; % measurement with measurement and process noise
% y = [zeros(3) Y_s]*xk + mk + v_k; % measurement with measurement and process noise
y = [zeros(3) Y_s]*xk; % measurement with no noise

== matlab function attempt_2_Full_Microthruster_Simulation/Sun Sensor Measurement Function/MATLAB Function ==
  data: xk input; y output; start_time input; sim_time input; sigma_s input; sigma_q input
function y = h(xk,start_time,sim_time,sigma_s,sigma_q)

% Start time is initial juliandate
% Sim time is current sim time in seconds

JD_new = start_time + sim_time/3600/24; % add sim time in days to start time

q = xk(4:7);
eps = q(1:3);
eta = q(4);

jul_cent = (JD_new-2451545)/36525; % julian centuries since 2000
lambda_S = wrapTo360(280.4606184 + 36000.77005361*jul_cent); % mean longitude of sun in deg
M_S = wrapTo360(357.5277233 + 35999.05034*jul_cent); % mean anomaly of sun in deg
lambda_e = wrapTo180(lambda_S + 1.914666471*sind(M_S) + 0.019994643*sind(2*M_S)); % ecliptic long of sun in deg

eps_sun = 23.439291-0.0130042*jul_cent;
sun_ECI = [cosd(lambda_e); cosd(eps_sun)*sind(lambda_e); sind(eps_sun)*sind(lambda_e)];

% Test for comparison
%sun_ECI = [1;0;0];
% Calculate Y(a,q) for magnetometer and sun sensor
% Y_b = [eta*eye(3)-Functions.vec2cross(eps) -eps]*[Functions.vec2cross(mag_ECI) mag_ECI;
%                                                       -mag_ECI'                    0];
Y_s = [eta*eye(3)-Functions.vec2cross(eps) -eps]*[Functions.vec2cross(sun_ECI) sun_ECI;
                                                      -sun_ECI'                    0];

coder.extrinsic('randn');
v_k = zeros([3 1]); %#ok<*PREALL> simulink needs this to determine variable size
v_k = randn(3,1)*sigma_q;   
m_k = zeros([3 1]);
m_k = randn(3,1)*sigma_s;
% y = [zeros(3) Y_s]*xk + m_k + v_k; % measurement with measurement and process noise
% y = [zeros(3) Y_s]*xk + mk + v_k; % measurement with measurement and process noise
y = [zeros(3) Y_s]*xk; % measurement with no noise

== matlab function attempt_2_Full_Microthruster_Simulation/Orbital Motion Propagator/MATLAB Function1 ==
  data: w_LVLH_ECI input; q_LVLH_ECI input; dquats_LVLH_ECI output; omega_b_ECI input; dquats output; w_b_LVLH input; q_b_ECI input; q_b_LVLH input; dquats_b_LVLH output
function [dquats_LVLH_ECI,dquats,dquats_b_LVLH] = quats(w_LVLH_ECI,q_LVLH_ECI,omega_b_ECI,w_b_LVLH,q_b_ECI,q_b_LVLH)

% ECI to Body
eps = q_b_ECI(1:3,1);
eta = q_b_ECI(4,1);

epsilonDot = 0.5*(eta*eye(3)+Functions.vec2cross(eps))*omega_b_ECI;
etaDot = -0.5*eps'*omega_b_ECI;

% LVLH to Body
eps_b_LVLH = q_b_LVLH(1:3);
eta_b_LVLH = q_b_LVLH(4);
epsilonDot_b_LVLH = 0.5*(eta_b_LVLH*eye(3)+Functions.vec2cross(eps_b_LVLH))*w_b_LVLH;
etaDot_b_LVLH = -0.5*eps_b_LVLH'*w_b_LVLH;

% ECI to LVLH
eps_LVLH_ECI = q_LVLH_ECI(1:3);
eta_LVLH_ECI = q_LVLH_ECI(4);
epsilonDot_LVLH_ECI = 0.5*(eta_LVLH_ECI*eye(3)+Functions.vec2cross(eps_LVLH_ECI))*w_LVLH_ECI;
etaDot_LVLH_ECI = -0.5*eps_LVLH_ECI'*w_LVLH_ECI;

dquats = [epsilonDot; etaDot];
dquats_b_LVLH = [epsilonDot_b_LVLH; etaDot_b_LVLH];
dquats_LVLH_ECI = [epsilonDot_LVLH_ECI; etaDot_LVLH_ECI];

== matlab function attempt_2_Full_Microthruster_Simulation/Orbital Motion Propagator/MATLAB Function2 ==
  data: E input; omega input; dE output; E_b_LVLH input; w_b_LVLH input; dE_b_LVLH output; E_LVLH_ECI input; w_LVLH_ECI input; dE_LVLH_ECI output
function [dE,dE_b_LVLH,dE_LVLH_ECI]  = euler(E,omega,E_b_LVLH,w_b_LVLH,E_LVLH_ECI,w_LVLH_ECI)

% ECI to Body
place = 1/cos(E(2))* [cos(E(2)) sin(E(1))*sin(E(2)) cos(E(1))*sin(E(2)); 
                        0          cos(E(1))*cos(E(2)) -sin(E(1))*cos(E(2)); 
                        0          sin(E(1))                  cos(E(1))];

dE =place*omega;

% LVLH to Body
place_b_LVLH = 1/cos(E_b_LVLH(2))* [cos(E_b_LVLH(2)) sin(E_b_LVLH(1))*sin(E_b_LVLH(2)) cos(E_b_LVLH(1))*sin(E_b_LVLH(2)); 
                        0          cos(E_b_LVLH(1))*cos(E_b_LVLH(2)) -sin(E_b_LVLH(1))*cos(E_b_LVLH(2)); 
                        0          sin(E_b_LVLH(1))                  cos(E_b_LVLH(1))];

dE_b_LVLH =place_b_LVLH*w_b_LVLH;

% ECI to LVLH
place_LVLH_ECI = 1/cos(E_LVLH_ECI(2))* [cos(E_LVLH_ECI(2)) sin(E_LVLH_ECI(1))*sin(E_LVLH_ECI(2)) cos(E_LVLH_ECI(1))*sin(E_LVLH_ECI(2)); 
                        0          cos(E_LVLH_ECI(1))*cos(E_LVLH_ECI(2)) -sin(E_LVLH_ECI(1))*cos(E_LVLH_ECI(2)); 
                        0          sin(E_LVLH_ECI(1))                  cos(E_LVLH_ECI(1))];

dE_LVLH_ECI =place_LVLH_ECI*w_LVLH_ECI;

== matlab function attempt_2_Full_Microthruster_Simulation/Orbital Motion Propagator/MATLAB Function3 ==
  data: rvec input; rdot output; vvec input; u input; vdot output
function [rdot,vdot] = rvProp(rvec,vvec,u)

rmag = norm(rvec);

% Calculate period in seconds and mean motion in rad/s
% T = 2*pi/sqrt(u)*(a)^(3/2); 
% n = 2*pi/T;
% Modify output to return mean motion if necessary

rdot = vvec;
vdot = -u*rvec/(rmag^3);

end

== matlab function attempt_2_Full_Microthruster_Simulation/Torque Vector Rotation ==
  data: q_b_ECI input; T_b input; T_ECI output; Tp_b input; Tp_ECI output
function [T_ECI,Tp_ECI] = fcn(q_b_ECI,T_b,Tp_b)
% Output constant thrust vector in ECI frame to correspond to dynamics
% model
q_b_ECI = q_b_ECI(4:7);
% Turn given ECI to Body quaternion into a rotation matrix
C_b_ECI = Functions.quat2rot(q_b_ECI);
C_ECI_b = C_b_ECI'; % Get Body to ECI rot matrix by transposing

T_ECI = C_ECI_b*T_b;
Tp_ECI = C_ECI_b*Tp_b;

== matlab function attempt_2_Full_Microthruster_Simulation/Orbital Motion Propagator/MATLAB Function4 ==
  data: q_LVLH_ECI input; r input; w_b_LVLH output; v input; omega input; w_LVLH_ECI output
function [w_b_LVLH,w_LVLH_ECI] = omega_b_LVLH(q_LVLH_ECI,r,v,omega)
C_LVLH_ECI = Functions.quat2rot(q_LVLH_ECI);
w_LVLH_ECI = C_LVLH_ECI*(cross(r,v)/norm(r)^2); % apply ECI to LVLH transformation matrix
w_b_LVLH = omega - w_LVLH_ECI;

% possibly needs rotation matrix
